simulink library "DSP_FPGA_Accelerated_Toolbox"  (R2019b)
settings: Solver=VariableStepAuto  StartTime=0.0  StopTime=10.0  RelTol=1e-3
undefined symbols (not defined in the file or in its folder): a, b, c
libraries: hdlsllib x54, simulink x17, $bdroot x2, dsphdlfiltering x1
(part 2 of 2)

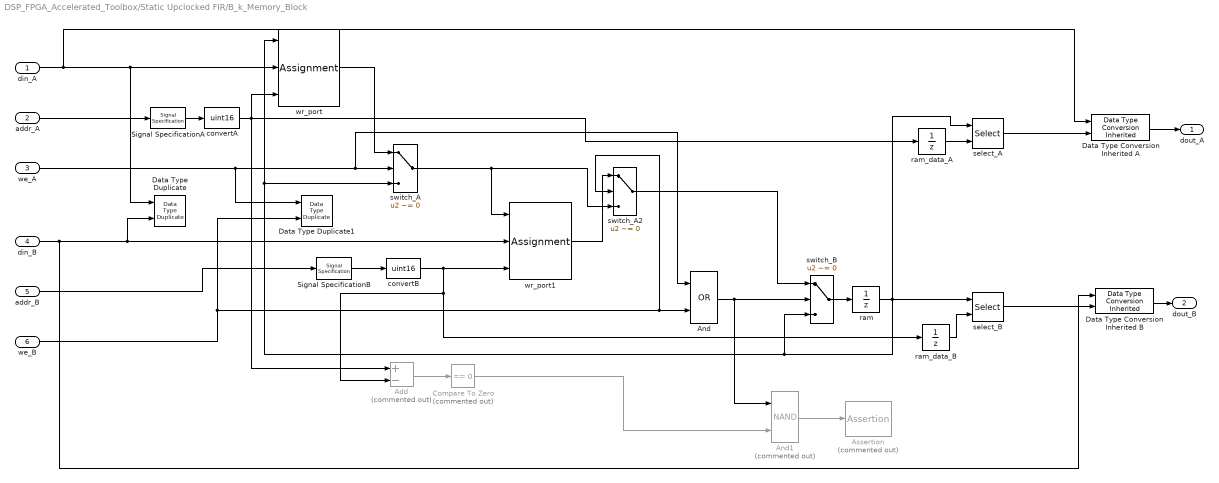
== system DSP_FPGA_Accelerated_Toolbox/Static Upclocked FIR/B_k_Memory_Block ==
  din_A : Inport
  addr_A : Inport  Port=2
  we_A : Inport  Port=3  OutDataTypeStr=boolean
  din_B : Inport  Port=4
  addr_B : Inport  Port=5
  we_B : Inport  Port=6  OutDataTypeStr=boolean
  Add : Sum  Commented=on  Inputs=+-
  And : Logic  Operator=OR  AllPortsSameDT=off  OutDataTypeStr=boolean
  And1 : Logic  Commented=on  Operator=NAND  AllPortsSameDT=off  OutDataTypeStr=boolean
  Assertion : Assertion  Commented=on  StopWhenAssertionFail=off
  Compare To Zero : simulink/Logic and Bit Operations/Compare To Zero  Commented=on  relop===  OutDataTypeStr=boolean
  Data Type Conversion Inherited A : simulink/Signal Attributes/Data Type Conversion Inherited  ConvertRealWorld=Real World Value  DoSatur=off
      settings: SourceProductName=Simulink  SourceProductBaseCode=SL
  Data Type Conversion Inherited B : simulink/Signal Attributes/Data Type Conversion Inherited  ConvertRealWorld=Real World Value  DoSatur=off
      settings: SourceProductName=Simulink  SourceProductBaseCode=SL
  Data Type Duplicate : DataTypeDuplicate
  Data Type Duplicate1 : DataTypeDuplicate
  Signal SpecificationA : SignalSpecification  OutDataTypeStr=fixdt(0,ram_size,0)  Dimensions=1
  Signal SpecificationB : SignalSpecification  OutDataTypeStr=fixdt(0,ram_size,0)  Dimensions=1
  convertA : DataTypeConversion  OutDataTypeStr=uint16
  convertB : DataTypeConversion  OutDataTypeStr=uint16
  ram : UnitDelay  InitialCondition=B_k_init  SampleTime=-1  HasFrameUpgradeWarning=on
  ram_data_A : UnitDelay  SampleTime=-1  HasFrameUpgradeWarning=on
  ram_data_B : UnitDelay  SampleTime=-1  HasFrameUpgradeWarning=on
  select_A : Selector  IndexMode=Zero-based  InputPortWidth=2^ram_size  IndexOptions=Index vector (port)  Indices=[1 3]  OutputSizes=1
  select_B : Selector  IndexMode=Zero-based  InputPortWidth=2^ram_size  IndexOptions=Index vector (port)  Indices=[1 3]  OutputSizes=1
  switch_A : Switch  Criteria=u2 ~= 0
  switch_A2 : Switch  Criteria=u2 ~= 0
  switch_B : Switch  Criteria=u2 ~= 0
  wr_port : Assignment  IndexMode=Zero-based  IndexOptions=Index vector (port)  Indices=1  OutputSizes=[1 1]
  wr_port1 : Assignment  IndexMode=Zero-based  IndexOptions=Index vector (port)  Indices=1  OutputSizes=[1 1]
  dout_A : Outport  VectorParamsAs1DForOutWhenUnconnected=off
  dout_B : Outport  Port=2  VectorParamsAs1DForOutWhenUnconnected=off
  wires:
  switch_A2/1 -> switch_B/1
  And1/1 -> Assertion/1
  Signal SpecificationA/1 -> convertA/1
  Signal SpecificationB/1 -> convertB/1
  switch_B/1 -> ram/1
  convertA/1 -> ram_data_A/1, wr_port/3, Add/1
  ram/1 -> select_B/1, switch_B/3, switch_A/3, wr_port/1, select_A/1
  wr_port/1 -> switch_A/1
  And/1 -> And1/1, switch_B/2
  wr_port1/1 -> switch_A2/1
  Add/1 -> Compare To Zero/1
  Compare To Zero/1 -> And1/2
  we_B/1 -> switch_A2/2, And/2, Data Type Duplicate1/2
  switch_A/1 -> wr_port1/1, switch_A2/3
  addr_B/1 -> Signal SpecificationB/1
  ram_data_B/1 -> select_B/2
  we_A/1 -> Data Type Duplicate1/1, And/1, switch_A/2
  ram_data_A/1 -> select_A/2
  din_A/1 -> Data Type Duplicate/1, wr_port/2, Data Type Conversion Inherited A/1
  convertB/1 -> ram_data_B/1, Add/2, wr_port1/3
  din_B/1 -> wr_port1/2, Data Type Duplicate/2, Data Type Conversion Inherited B/1
  addr_A/1 -> Signal SpecificationA/1
  select_B/1 -> Data Type Conversion Inherited B/2
  Data Type Conversion Inherited B/1 -> dout_B/1
  select_A/1 -> Data Type Conversion Inherited A/2
  Data Type Conversion Inherited A/1 -> dout_A/1

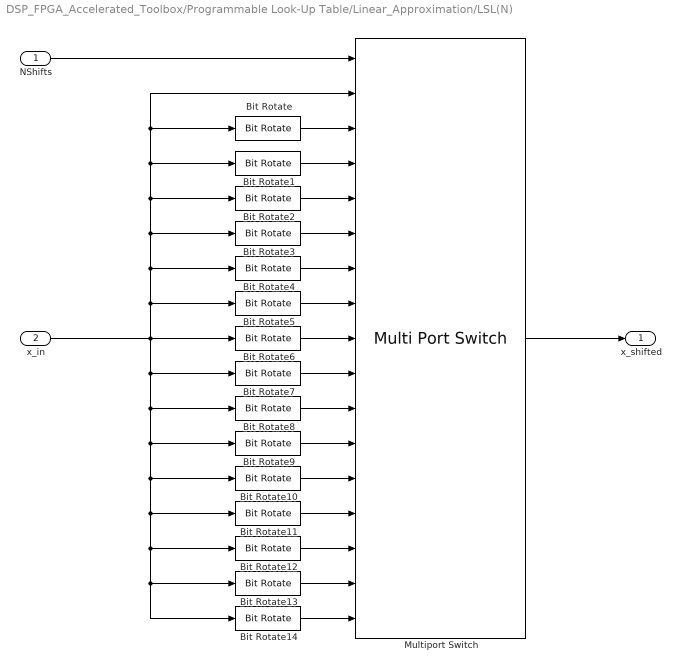
== system DSP_FPGA_Accelerated_Toolbox/Programmable Look-Up Table/Linear_Approximation/LSL(N) ==
  NShifts : Inport
  x_in : Inport  Port=2
  Bit Rotate : hdlsllib/Logic and Bit Operations/Bit Rotate  mode=Rotate Left  N=1
      settings: SourceProductName=Simulink  SourceProductBaseCode=SL
  Bit Rotate1 : hdlsllib/Logic and Bit Operations/Bit Rotate  mode=Rotate Left  N=2
      settings: SourceProductName=Simulink  SourceProductBaseCode=SL
  Bit Rotate10 : hdlsllib/Logic and Bit Operations/Bit Rotate  mode=Rotate Left  N=11
      settings: SourceProductName=Simulink  SourceProductBaseCode=SL
  Bit Rotate11 : hdlsllib/Logic and Bit Operations/Bit Rotate  mode=Rotate Left  N=12
      settings: SourceProductName=Simulink  SourceProductBaseCode=SL
  Bit Rotate12 : hdlsllib/Logic and Bit Operations/Bit Rotate  mode=Rotate Left  N=13
      settings: SourceProductName=Simulink  SourceProductBaseCode=SL
  Bit Rotate13 : hdlsllib/Logic and Bit Operations/Bit Rotate  mode=Rotate Left  N=14
      settings: SourceProductName=Simulink  SourceProductBaseCode=SL
  Bit Rotate14 : hdlsllib/Logic and Bit Operations/Bit Rotate  mode=Rotate Left  N=15
      settings: SourceProductName=Simulink  SourceProductBaseCode=SL
  Bit Rotate2 : hdlsllib/Logic and Bit Operations/Bit Rotate  mode=Rotate Left  N=3
      settings: SourceProductName=Simulink  SourceProductBaseCode=SL
  Bit Rotate3 : hdlsllib/Logic and Bit Operations/Bit Rotate  mode=Rotate Left  N=4
      settings: SourceProductName=Simulink  SourceProductBaseCode=SL
  Bit Rotate4 : hdlsllib/Logic and Bit Operations/Bit Rotate  mode=Rotate Left  N=5
      settings: SourceProductName=Simulink  SourceProductBaseCode=SL
  Bit Rotate5 : hdlsllib/Logic and Bit Operations/Bit Rotate  mode=Rotate Left  N=6
      settings: SourceProductName=Simulink  SourceProductBaseCode=SL
  Bit Rotate6 : hdlsllib/Logic and Bit Operations/Bit Rotate  mode=Rotate Left  N=7
      settings: SourceProductName=Simulink  SourceProductBaseCode=SL
  Bit Rotate7 : hdlsllib/Logic and Bit Operations/Bit Rotate  mode=Rotate Left  N=8
      settings: SourceProductName=Simulink  SourceProductBaseCode=SL
  Bit Rotate8 : hdlsllib/Logic and Bit Operations/Bit Rotate  mode=Rotate Left  N=9
      settings: SourceProductName=Simulink  SourceProductBaseCode=SL
  Bit Rotate9 : hdlsllib/Logic and Bit Operations/Bit Rotate  mode=Rotate Left  N=10
      settings: SourceProductName=Simulink  SourceProductBaseCode=SL
  Multiport Switch : MultiPortSwitch  DataPortOrder=Zero-based contiguous  Inputs=16  DiagnosticForDefault=Warning  zeroidx=on
  x_shifted : Outport  VectorParamsAs1DForOutWhenUnconnected=off
  wires:
  NShifts/1 -> Multiport Switch/1
  Multiport Switch/1 -> x_shifted/1
  x_in/1 -> Bit Rotate12/1, Bit Rotate13/1, Bit Rotate14/1, Bit Rotate11/1, Bit Rotate10/1, Bit Rotate9/1, Bit Rotate8/1, Bit Rotate7/1, Bit Rotate5/1, Bit Rotate4/1, Multiport Switch/2, Bit Rotate/1, Bit Rotate1/1, Bit Rotate2/1, Bit Rotate3/1, Bit Rotate6/1
  Bit Rotate/1 -> Multiport Switch/3
  Bit Rotate1/1 -> Multiport Switch/4
  Bit Rotate2/1 -> Multiport Switch/5
  Bit Rotate3/1 -> Multiport Switch/6
  Bit Rotate4/1 -> Multiport Switch/7
  Bit Rotate5/1 -> Multiport Switch/8
  Bit Rotate6/1 -> Multiport Switch/9
  Bit Rotate7/1 -> Multiport Switch/10
  Bit Rotate8/1 -> Multiport Switch/11
  Bit Rotate9/1 -> Multiport Switch/12
  Bit Rotate10/1 -> Multiport Switch/13
  Bit Rotate11/1 -> Multiport Switch/14
  Bit Rotate12/1 -> Multiport Switch/15
  Bit Rotate13/1 -> Multiport Switch/16
  Bit Rotate14/1 -> Multiport Switch/17

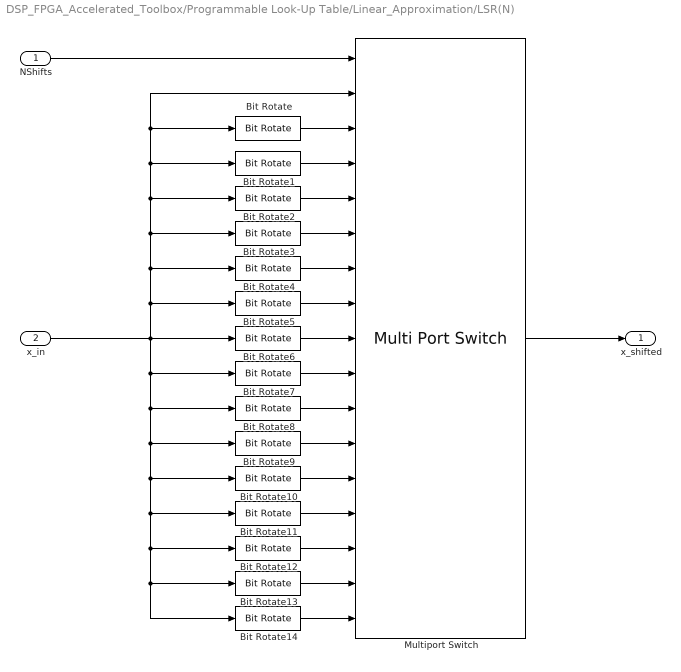
== system DSP_FPGA_Accelerated_Toolbox/Programmable Look-Up Table/Linear_Approximation/LSR(N) ==
  NShifts : Inport
  x_in : Inport  Port=2
  Bit Rotate : hdlsllib/Logic and Bit Operations/Bit Rotate  mode=Rotate Right  N=1
      settings: SourceProductName=Simulink  SourceProductBaseCode=SL
  Bit Rotate1 : hdlsllib/Logic and Bit Operations/Bit Rotate  mode=Rotate Right  N=2
      settings: SourceProductName=Simulink  SourceProductBaseCode=SL
  Bit Rotate10 : hdlsllib/Logic and Bit Operations/Bit Rotate  mode=Rotate Right  N=11
      settings: SourceProductName=Simulink  SourceProductBaseCode=SL
  Bit Rotate11 : hdlsllib/Logic and Bit Operations/Bit Rotate  mode=Rotate Right  N=12
      settings: SourceProductName=Simulink  SourceProductBaseCode=SL
  Bit Rotate12 : hdlsllib/Logic and Bit Operations/Bit Rotate  mode=Rotate Right  N=13
      settings: SourceProductName=Simulink  SourceProductBaseCode=SL
  Bit Rotate13 : hdlsllib/Logic and Bit Operations/Bit Rotate  mode=Rotate Right  N=14
      settings: SourceProductName=Simulink  SourceProductBaseCode=SL
  Bit Rotate14 : hdlsllib/Logic and Bit Operations/Bit Rotate  mode=Rotate Right  N=15
      settings: SourceProductName=Simulink  SourceProductBaseCode=SL
  Bit Rotate2 : hdlsllib/Logic and Bit Operations/Bit Rotate  mode=Rotate Right  N=3
      settings: SourceProductName=Simulink  SourceProductBaseCode=SL
  Bit Rotate3 : hdlsllib/Logic and Bit Operations/Bit Rotate  mode=Rotate Right  N=4
      settings: SourceProductName=Simulink  SourceProductBaseCode=SL
  Bit Rotate4 : hdlsllib/Logic and Bit Operations/Bit Rotate  mode=Rotate Right  N=5
      settings: SourceProductName=Simulink  SourceProductBaseCode=SL
  Bit Rotate5 : hdlsllib/Logic and Bit Operations/Bit Rotate  mode=Rotate Right  N=6
      settings: SourceProductName=Simulink  SourceProductBaseCode=SL
  Bit Rotate6 : hdlsllib/Logic and Bit Operations/Bit Rotate  mode=Rotate Right  N=7
      settings: SourceProductName=Simulink  SourceProductBaseCode=SL
  Bit Rotate7 : hdlsllib/Logic and Bit Operations/Bit Rotate  mode=Rotate Right  N=8
      settings: SourceProductName=Simulink  SourceProductBaseCode=SL
  Bit Rotate8 : hdlsllib/Logic and Bit Operations/Bit Rotate  mode=Rotate Right  N=9
      settings: SourceProductName=Simulink  SourceProductBaseCode=SL
  Bit Rotate9 : hdlsllib/Logic and Bit Operations/Bit Rotate  mode=Rotate Right  N=10
      settings: SourceProductName=Simulink  SourceProductBaseCode=SL
  Multiport Switch : MultiPortSwitch  DataPortOrder=Zero-based contiguous  Inputs=16  DiagnosticForDefault=Warning  zeroidx=on
  x_shifted : Outport  VectorParamsAs1DForOutWhenUnconnected=off
  wires:
  NShifts/1 -> Multiport Switch/1
  Multiport Switch/1 -> x_shifted/1
  x_in/1 -> Bit Rotate12/1, Bit Rotate13/1, Bit Rotate14/1, Bit Rotate11/1, Bit Rotate10/1, Bit Rotate9/1, Bit Rotate8/1, Bit Rotate7/1, Bit Rotate5/1, Bit Rotate4/1, Multiport Switch/2, Bit Rotate/1, Bit Rotate1/1, Bit Rotate2/1, Bit Rotate3/1, Bit Rotate6/1
  Bit Rotate/1 -> Multiport Switch/3
  Bit Rotate1/1 -> Multiport Switch/4
  Bit Rotate2/1 -> Multiport Switch/5
  Bit Rotate3/1 -> Multiport Switch/6
  Bit Rotate4/1 -> Multiport Switch/7
  Bit Rotate5/1 -> Multiport Switch/8
  Bit Rotate6/1 -> Multiport Switch/9
  Bit Rotate7/1 -> Multiport Switch/10
  Bit Rotate8/1 -> Multiport Switch/11
  Bit Rotate9/1 -> Multiport Switch/12
  Bit Rotate10/1 -> Multiport Switch/13
  Bit Rotate11/1 -> Multiport Switch/14
  Bit Rotate12/1 -> Multiport Switch/15
  Bit Rotate13/1 -> Multiport Switch/16
  Bit Rotate14/1 -> Multiport Switch/17

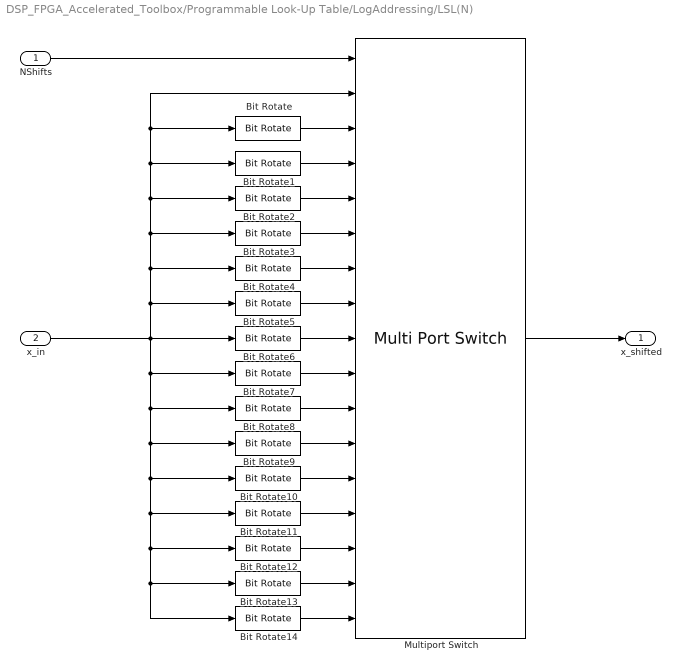
== system DSP_FPGA_Accelerated_Toolbox/Programmable Look-Up Table/LogAddressing/LSL(N) ==
  NShifts : Inport
  x_in : Inport  Port=2
  Bit Rotate : hdlsllib/Logic and Bit Operations/Bit Rotate  mode=Rotate Left  N=1
      settings: SourceProductName=Simulink  SourceProductBaseCode=SL
  Bit Rotate1 : hdlsllib/Logic and Bit Operations/Bit Rotate  mode=Rotate Left  N=2
      settings: SourceProductName=Simulink  SourceProductBaseCode=SL
  Bit Rotate10 : hdlsllib/Logic and Bit Operations/Bit Rotate  mode=Rotate Left  N=11
      settings: SourceProductName=Simulink  SourceProductBaseCode=SL
  Bit Rotate11 : hdlsllib/Logic and Bit Operations/Bit Rotate  mode=Rotate Left  N=12
      settings: SourceProductName=Simulink  SourceProductBaseCode=SL
  Bit Rotate12 : hdlsllib/Logic and Bit Operations/Bit Rotate  mode=Rotate Left  N=13
      settings: SourceProductName=Simulink  SourceProductBaseCode=SL
  Bit Rotate13 : hdlsllib/Logic and Bit Operations/Bit Rotate  mode=Rotate Left  N=14
      settings: SourceProductName=Simulink  SourceProductBaseCode=SL
  Bit Rotate14 : hdlsllib/Logic and Bit Operations/Bit Rotate  mode=Rotate Left  N=15
      settings: SourceProductName=Simulink  SourceProductBaseCode=SL
  Bit Rotate2 : hdlsllib/Logic and Bit Operations/Bit Rotate  mode=Rotate Left  N=3
      settings: SourceProductName=Simulink  SourceProductBaseCode=SL
  Bit Rotate3 : hdlsllib/Logic and Bit Operations/Bit Rotate  mode=Rotate Left  N=4
      settings: SourceProductName=Simulink  SourceProductBaseCode=SL
  Bit Rotate4 : hdlsllib/Logic and Bit Operations/Bit Rotate  mode=Rotate Left  N=5
      settings: SourceProductName=Simulink  SourceProductBaseCode=SL
  Bit Rotate5 : hdlsllib/Logic and Bit Operations/Bit Rotate  mode=Rotate Left  N=6
      settings: SourceProductName=Simulink  SourceProductBaseCode=SL
  Bit Rotate6 : hdlsllib/Logic and Bit Operations/Bit Rotate  mode=Rotate Left  N=7
      settings: SourceProductName=Simulink  SourceProductBaseCode=SL
  Bit Rotate7 : hdlsllib/Logic and Bit Operations/Bit Rotate  mode=Rotate Left  N=8
      settings: SourceProductName=Simulink  SourceProductBaseCode=SL
  Bit Rotate8 : hdlsllib/Logic and Bit Operations/Bit Rotate  mode=Rotate Left  N=9
      settings: SourceProductName=Simulink  SourceProductBaseCode=SL
  Bit Rotate9 : hdlsllib/Logic and Bit Operations/Bit Rotate  mode=Rotate Left  N=10
      settings: SourceProductName=Simulink  SourceProductBaseCode=SL
  Multiport Switch : MultiPortSwitch  DataPortOrder=Zero-based contiguous  Inputs=16  DiagnosticForDefault=Warning  zeroidx=on
  x_shifted : Outport  VectorParamsAs1DForOutWhenUnconnected=off
  wires:
  NShifts/1 -> Multiport Switch/1
  Multiport Switch/1 -> x_shifted/1
  x_in/1 -> Bit Rotate12/1, Bit Rotate13/1, Bit Rotate14/1, Bit Rotate11/1, Bit Rotate10/1, Bit Rotate9/1, Bit Rotate8/1, Bit Rotate7/1, Bit Rotate5/1, Bit Rotate4/1, Multiport Switch/2, Bit Rotate/1, Bit Rotate1/1, Bit Rotate2/1, Bit Rotate3/1, Bit Rotate6/1
  Bit Rotate/1 -> Multiport Switch/3
  Bit Rotate1/1 -> Multiport Switch/4
  Bit Rotate2/1 -> Multiport Switch/5
  Bit Rotate3/1 -> Multiport Switch/6
  Bit Rotate4/1 -> Multiport Switch/7
  Bit Rotate5/1 -> Multiport Switch/8
  Bit Rotate6/1 -> Multiport Switch/9
  Bit Rotate7/1 -> Multiport Switch/10
  Bit Rotate8/1 -> Multiport Switch/11
  Bit Rotate9/1 -> Multiport Switch/12
  Bit Rotate10/1 -> Multiport Switch/13
  Bit Rotate11/1 -> Multiport Switch/14
  Bit Rotate12/1 -> Multiport Switch/15
  Bit Rotate13/1 -> Multiport Switch/16
  Bit Rotate14/1 -> Multiport Switch/17

== matlab function DSP_FPGA_Accelerated_Toolbox/Programmable Look-Up Table/LogAddressing/MATLAB Function ==
  data: x input; lzc_count output
function lzc_count = fcn(x)
%#codegen

% -- Binary Bisection Tree (Divide & Conquer)
if bitorreduce(x, 40, 21) == 1 %       if ((b39 or b38 or b37 or b36 or b35 or b34 or b33 or b32 or b31 or b30 or b29 or b28 or b27 or b26 or b25 or b24 or b23 or b22 or b21 or b20) = '1') then   -- check bit range [39  20]
    if bitorreduce(x, 40, 31) == 1%             if ((b39 or b38 or b37 or b36 or b35 or b34 or b33 or b32 or b31 or b30) = '1') then   -- check bit range [39  30]
        if bitorreduce(x, 40, 36) == 1%                 if ((b39 or b38 or b37 or b36 or b35) = '1') then   -- check bit range [39  35]
            if bitorreduce(x, 40, 38) == 1%                     if ((b39 or b38 or b37) = '1') then   -- check bit range [39  37]
                if bitorreduce(x, 40, 39) == 1%                         if ((b39 or b38) = '1') then   -- check bit range [39  38]
                    if bitorreduce(x, 40, 40) == 1%                             if (b39 = '1') then   -- [39]
                        lzc_count = fi(0,0,6,0);%                                 lzc_count <= "000000";  -- lzc = 0
                    else%                             else  -- check bit range [38]
                        lzc_count = fi(1,0,6,0);%                                 lzc_count <= "000001";  -- lzc = 1
                    end%                             end if;
                else%                         else  -- check bit range [37]
                    lzc_count = fi(2,0,6,0);%                             lzc_count <= "000010";  -- lzc = 2
                end%                         end if;
            else%                     else  -- check bit range [36  35]
                if bitorreduce(x, 37, 37) == 1%                         if (b36 = '1') then   -- [36]
                    lzc_count = fi(3,0,6,0);%                             lzc_count <= "000011";  -- lzc = 3
                else%                         else  -- check bit range [35]
                    lzc_count = fi(4,0,6,0);%                             lzc_count <= "000100";  -- lzc = 4
                end%                         end if;
            end%                     end if;
        else%                 else  -- check bit range [34  30]
            if bitorreduce(x, 35, 33) == 1%                     if ((b34 or b33 or b32) = '1') then   -- check bit range [34  32]
                if bitorreduce(x, 35, 34) == 1%                         if ((b34 or b33) = '1') then   -- check bit range [34  33]
                    if bitorreduce(x, 35, 35) == 1%                             if (b34 = '1') then   -- [34]
                        lzc_count = fi(5,0,6,0);%                                 lzc_count <= "000101";  -- lzc = 5
                    else%                             else  -- check bit range [33]
                        lzc_count = fi(6,0,6,0);%                                 lzc_count <= "000110";  -- lzc = 6
                    end%                             end if;
                else%                         else  -- check bit range [32]
                    lzc_count = fi(7,0,6,0);%                             lzc_count <= "000111";  -- lzc = 7
                end%                         end if;
            else%                     else  -- check bit range [31  30]
                if bitorreduce(x, 32, 32) == 1%                         if (b31 = '1') then   -- [31]
                    lzc_count = fi(8,0,6,0);%                             lzc_count <= "001000";  -- lzc = 8
                else%                         else  -- check bit range [30]
                    lzc_count = fi(9,0,6,0);%                             lzc_count <= "001001";  -- lzc = 9
                end%                         end if;
            end%                     end if;
        end%                 end if;
    else%             else  -- check bit range [29  20]
        if bitorreduce(x, 30, 26) == 1%                 if ((b29 or b28 or b27 or b26 or b25) = '1') then   -- check bit range [29  25]
            if bitorreduce(x, 30, 28) == 1%                     if ((b29 or b28 or b27) = '1') then   -- check bit range [29  27]
                if bitorreduce(x, 30, 29) == 1%                         if ((b29 or b28) = '1') then   -- check bit range [29  28]
                    if bitorreduce(x, 30, 30) == 1%                             if (b29 = '1') then   -- [29]
                        lzc_count = fi(10,0,6,0);%                                 lzc_count <= "001010";  -- lzc = 10
                    else%                             else  -- check bit range [28]
                        lzc_count = fi(11,0,6,0);%                                 lzc_count <= "001011";  -- lzc = 11
                    end%                             end if;
                else%                         else  -- check bit range [27]
                    lzc_count = fi(12,0,6,0);%                             lzc_count <= "001100";  -- lzc = 12
                end%                         end if;
            else%                     else  -- check bit range [26  25]
                if bitorreduce(x, 27, 27) == 1%                         if (b26 = '1') then   -- [26]
                    lzc_count = fi(13,0,6,0);%                             lzc_count <= "001101";  -- lzc = 13
                else%                         else  -- check bit range [25]
                    lzc_count = fi(14,0,6,0);%                             lzc_count <= "001110";  -- lzc = 14
                end%                         end if;
            end%                     end if;
        else%                 else  -- check bit range [24  20]
            if bitorreduce(x, 25, 23) == 1%                     if ((b24 or b23 or b22) = '1') then   -- check bit range [24  22]
                if bitorreduce(x, 25, 24) == 1%                         if ((b24 or b23) = '1') then   -- check bit range [24  23]
                    if bitorreduce(x, 25, 25) == 1%                             if (b24 = '1') then   -- [24]
                        lzc_count = fi(15,0,6,0);%                                 lzc_count <= "001111";  -- lzc = 15
                    else%                             else  -- check bit range [23]
                        lzc_count = fi(16,0,6,0);%                                 lzc_count <= "010000";  -- lzc = 16
                    end%                             end if;
                else%                         else  -- check bit range [22]
                    lzc_count = fi(17,0,6,0);%                             lzc_count <= "010001";  -- lzc = 17
                end%                         end if;
            else%                     else  -- check bit range [21  20]
                if bitorreduce(x, 22, 22) == 1%                         if (b21 = '1') then   -- [21]
                    lzc_count = fi(18,0,6,0);%                             lzc_count <= "010010";  -- lzc = 18
                else%                         else  -- check bit range [20]
                    lzc_count = fi(19,0,6,0);%                             lzc_count <= "010011";  -- lzc = 19
                end%                         end if;
            end%                     end if;
        end%                 end if;
    end%             end if;
else%         else  -- check bit range [19   0]
    if bitorreduce(x, 20, 11) == 1%             if ((b19 or b18 or b17 or b16 or b15 or b14 or b13 or b12 or b11 or b10) = '1') then   -- check bit range [19  10]
        if bitorreduce(x, 20, 16) == 1%                 if ((b19 or b18 or b17 or b16 or b15) = '1') then   -- check bit range [19  15]
            if bitorreduce(x, 20, 18) == 1%                     if ((b19 or b18 or b17) = '1') then   -- check bit range [19  17]
                if bitorreduce(x, 20, 19) == 1%                         if ((b19 or b18) = '1') then   -- check bit range [19  18]
                    if bitorreduce(x, 20, 20) == 1%                             if (b19 = '1') then   -- [19]
                        lzc_count = fi(20,0,6,0);%                                 lzc_count <= "010100";  -- lzc = 20
                    else%                             else  -- check bit range [18]
                        lzc_count = fi(21,0,6,0);%                                 lzc_count <= "010101";  -- lzc = 21
                    end%                             end if;
                else%                         else  -- check bit range [17]
                    lzc_count = fi(22,0,6,0);%                             lzc_count <= "010110";  -- lzc = 22
                end%                         end if;
            else%                     else  -- check bit range [16  15]
                if bitorreduce(x, 17, 17) == 1%                         if (b16 = '1') then   -- [16]
                    lzc_count = fi(23,0,6,0);%                             lzc_count <= "010111";  -- lzc = 23
                else%                         else  -- check bit range [15]
                    lzc_count = fi(24,0,6,0);%                             lzc_count <= "011000";  -- lzc = 24
                end%                         end if;
            end%                     end if;
        else%                 else  -- check bit range [14  10]
            if bitorreduce(x, 15, 13) == 1%                     if ((b14 or b13 or b12) = '1') then   -- check bit range [14  12]
                if bitorreduce(x, 15, 14) == 1%                         if ((b14 or b13) = '1') then   -- check bit range [14  13]
                    if bitorreduce(x, 15, 15) == 1%                             if (b14 = '1') then   -- [14]
                        lzc_count = fi(25,0,6,0);%                                 lzc_count <= "011001";  -- lzc = 25
                    else%                             else  -- check bit range [13]
                        lzc_count = fi(26,0,6,0);%                                 lzc_count <= "011010";  -- lzc = 26
                    end%                             end if;
                else%                         else  -- check bit range [12]
                    lzc_count = fi(27,0,6,0);%                             lzc_count <= "011011";  -- lzc = 27
                end%                         end if;
            else%                     else  -- check bit range [11  10]
                if bitorreduce(x, 12, 12) == 1%                         if (b11 = '1') then   -- [11]
                    lzc_count = fi(28,0,6,0);%                             lzc_count <= "011100";  -- lzc = 28
                else%                         else  -- check bit range [10]
                    lzc_count = fi(29,0,6,0);%                             lzc_count <= "011101";  -- lzc = 29
                end%                         end if;
            end%                     end if;
        end%                 end if;
    else%             else  -- check bit range [9  0]
        if bitorreduce(x, 10, 6) == 1%                 if ((b9 or b8 or b7 or b6 or b5) = '1') then   -- check bit range [9  5]
            if bitorreduce(x, 10, 9) == 1%                     if ((b9 or b8 or b7) = '1') then   -- check bit range [9  7]
                if bitorreduce(x, 10, 9) == 1%                         if ((b9 or b8) = '1') then   -- check bit range [9  8]
                    if bitorreduce(x, 10, 10) == 1%                             if (b9 = '1') then   -- [9]
                        lzc_count = fi(30,0,6,0);%                                 lzc_count <= "011110";  -- lzc = 30
                    else%                             else  -- check bit range [8]
                        lzc_count = fi(31,0,6,0);%                                 lzc_count <= "011111";  -- lzc = 31
                    end%                             end if;
                else%                         else  -- check bit range [7]
                    lzc_count = fi(32,0,6,0);%                             lzc_count <= "100000";  -- lzc = 32
                end%                         end if;
            else%                     else  -- check bit range [6  5]
                if bitorreduce(x, 7, 7) == 1%                         if (b6 = '1') then   -- [6]
                    lzc_count = fi(33,0,6,0);%                             lzc_count <= "100001";  -- lzc = 33
                else%                         else  -- check bit range [5]
                    lzc_count = fi(34,0,6,0);%                             lzc_count <= "100010";  -- lzc = 34
                end%                         end if;
            end%                     end if;
        else%                 else  -- check bit range [4  0]
            if bitorreduce(x, 5, 3) == 1%                     if ((b4 or b3 or b2) = '1') then   -- check bit range [4  2]
                if bitorreduce(x, 5, 4) == 1%                         if ((b4 or b3) = '1') then   -- check bit range [4  3]
                    if bitorreduce(x, 5, 5) == 1%                             if (b4 = '1') then   -- [4]
                        lzc_count = fi(35,0,6,0);%                                 lzc_count <= "100011";  -- lzc = 35
                    else%                             else  -- check bit range [3]
                        lzc_count = fi(36,0,6,0);%                                 lzc_count <= "100100";  -- lzc = 36
                    end%                             end if;
                else%                         else  -- check bit range [2]
                    lzc_count = fi(37,0,6,0);%                             lzc_count <= "100101";  -- lzc = 37
                end%                         end if;
            else%                     else  -- check bit range [1  0]
                if bitorreduce(x, 2, 2) == 1%                         if (b1 = '1') then   -- [1]
                    lzc_count = fi(38,0,6,0);%                             lzc_count <= "100110";  -- lzc = 38
                else%                         else  -- check bit range [0]
                    lzc_count = fi(39,0,6,0);%                             lzc_count <= "100111";  -- lzc = 39
                end%                         end if;
            end%                     end if;
        end%                 end if;
    end%             end if;
end%         end if;
